simulink model "SERVO_DC_MOTOR"  (R2020a)
settings: Solver=VariableStepAuto  StartTime=0.0  StopTime=10.0  RelTol=1e-3
undefined symbols (not defined in the file): b, j, kb, kt, L, R
settings Model: Creator=naina  LastModifiedBy=naina

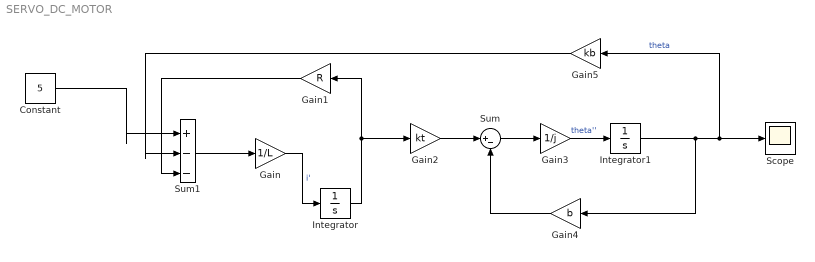
== system SERVO_DC_MOTOR ==
  Constant : Constant  Value=5
  Gain : Gain  Gain=1/L
  Gain1 : Gain  Gain=R
  Gain2 : Gain  Gain=kt
  Gain3 : Gain  Gain=1/j
  Gain4 : Gain  Gain=b
  Gain5 : Gain  Gain=kb
  Integrator : Integrator
  Integrator1 : Integrator
  Scope : Scope
  Sum : Sum  Inputs=|+-
  Sum1 : Sum  Inputs=|+--
  wires:
  Integrator/1 -> Gain1/1, Gain2/1
  Gain3/1 -> Integrator1/1  "theta''"
  Integrator1/1 -> Gain4/1, Gain5/1, Scope/1  "theta"
  Gain4/1 -> Sum/2
  Sum/1 -> Gain3/1
  Gain2/1 -> Sum/1
  Constant/1 -> Sum1/1
  Sum1/1 -> Gain/1
  Gain/1 -> Integrator/1  "i'"
  Gain5/1 -> Sum1/2
  Gain1/1 -> Sum1/3
